simulink model "chap04_01_02_mdl"  (R2013b)
settings: Solver=FixedStepDiscrete  StartTime=0.0  StopTime=10.0  RelTol=1e-3
settings Model: Creator=Administrator  LastModifiedBy=sunzx.fnst

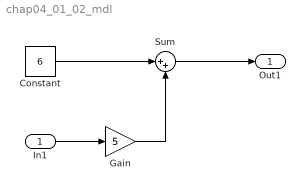
== system chap04_01_02_mdl ==
  In1 : Inport
  Constant : Constant  Value=6
  Gain : Gain  Gain=5
  Sum : Sum  Inputs=|++
  Out1 : Outport
  wires:
  In1/1 -> Gain/1
  Sum/1 -> Out1/1
  Constant/1 -> Sum/1
  Gain/1 -> Sum/2
